simulink model "FUZZY_tsc_neurospora_model_leloup"  (R2015a)
settings: Solver=ode4  StartTime=0.0  StopTime=72  FixedStep=0.01  RelTol=1e-3
values from neighbouring files (symbols this model uses):
  daynight_on = 0    [ALL_neurospora_init.m]    (also in ALL_neurospora_sim_run.m; FUZZY_deg_neurospora_init.m; FUZZY_deg_neurospora_sim_run.m; FUZZY_tsc_neurospora_init.m)
  k_1 = 0.5    [ALL_neurospora_init.m]    (also in FUZZY_deg_neurospora_init.m; FUZZY_tsc_neurospora_init.m; FUZZY_tsc_tsl_neurospora_init.m; FUZZY_tsl_neurospora_init.m)
  k_2 = 0.6    [ALL_neurospora_init.m]    (also in FUZZY_deg_neurospora_init.m; FUZZY_tsc_neurospora_init.m; FUZZY_tsc_tsl_neurospora_init.m; FUZZY_tsl_neurospora_init.m)
  K_d = 0.13    [ALL_neurospora_init.m]    (also in FUZZY_deg_neurospora_init.m; FUZZY_tsc_neurospora_init.m; FUZZY_tsc_tsl_neurospora_init.m; FUZZY_tsl_neurospora_init.m)
  K_m = 0.5    [ALL_neurospora_init.m]    (also in FUZZY_deg_neurospora_init.m; FUZZY_tsc_neurospora_init.m; FUZZY_tsc_tsl_neurospora_init.m; FUZZY_tsl_neurospora_init.m)
  k_s = 0.5    [ALL_neurospora_init.m]    (also in FUZZY_deg_neurospora_init.m; FUZZY_tsc_neurospora_init.m; FUZZY_tsc_tsl_neurospora_init.m; FUZZY_tsl_neurospora_init.m)
  v_d = 1.4    [ALL_neurospora_init.m]    (also in FUZZY_deg_neurospora_init.m; FUZZY_tsc_neurospora_init.m; FUZZY_tsc_tsl_neurospora_init.m; FUZZY_tsl_neurospora_init.m)
  v_m = 0.505    [ALL_neurospora_init.m]    (also in FUZZY_deg_neurospora_init.m; FUZZY_tsc_neurospora_init.m; FUZZY_tsc_tsl_neurospora_init.m; FUZZY_tsl_neurospora_init.m)
libraries: fuzblock x1
settings Model: Creator=jureb  LastModifiedBy=jureb

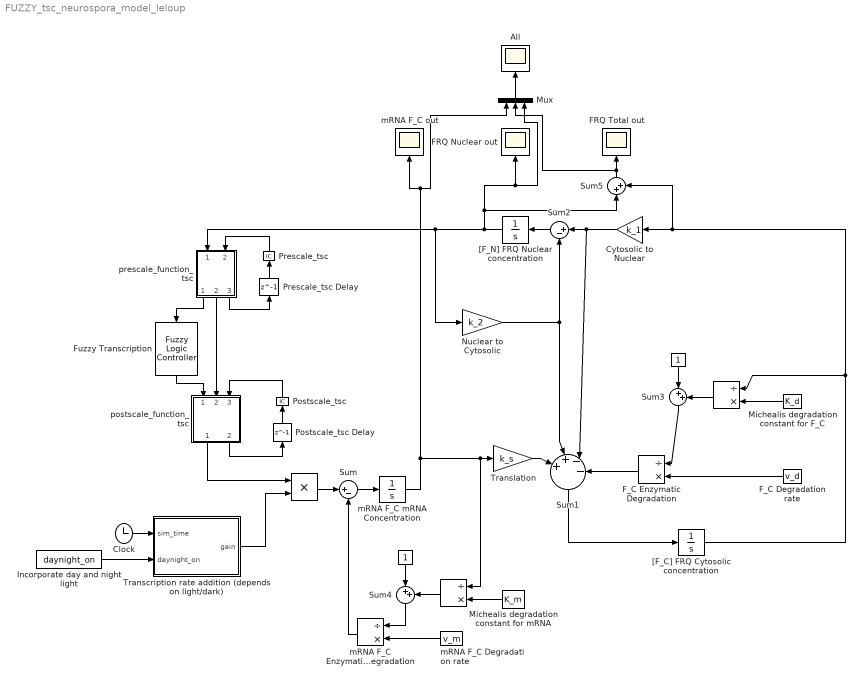
== system FUZZY_tsc_neurospora_model_leloup ==
  "    " : Product  Inputs=**
  " " : Product  Inputs=/*
  " " : Constant
  " " : Constant
  " " : Product  Inputs=/*
  All : Scope
      settings: TimeRange=71.999776  YMin=0  YMax=10  SaveName=All
  Clock : Clock
  Cytosolic to Nuclear : Gain  Gain=k_1
  FRQ Nuclear out : Scope
      settings: TimeRange=71.999776  YMin=0  YMax=4.5  SaveName=F_N
  FRQ Total out : Scope
      settings: TimeRange=71.999776  YMin=0.5  YMax=10  SaveName=F_FL_tsc
  F_C Degradation rate : Constant  Value=v_d
  F_C Enzymatic Degradation : Product  Inputs=/*
  Fuzzy Transcription : fuzblock/Fuzzy Logic  Controller  fis=tsc
  Incorporate day and night light : Constant  Value=daynight_on
  Michealis degradation constant for F_C : Constant  Value=K_d
  Michealis degradation constant for mRNA : Constant  Value=K_m
  Mux : Mux  Inputs=3
  Nuclear to Cytosolic : Gain  Gain=k_2
  Postscale_tsc : InitialCondition  Value=1.3
  Postscale_tsc Delay : Delay  DelayLength=1  InitialCondition=1
  Prescale_tsc : InitialCondition  Value=5
  Prescale_tsc Delay : Delay  DelayLength=1  InitialCondition=1  UseCircularBuffer=on
  Sum : Sum  Inputs=|+-
  Sum1 : Sum  Inputs=|+|+|-|-
  Sum2 : Sum  Inputs=|+-
  Sum3 : Sum  Inputs=|++
  Sum4 : Sum  Inputs=|++
  Sum5 : Sum  Inputs=|++
  Transcription rate addition (depends on light/dark) : MATLAB Function  TreatAsAtomicUnit=on
  Translation : Gain  Gain=k_s
  "[F_C] FRQ Cytosolic concentration " : Integrator  InitialCondition=1
  "[F_N] FRQ Nuclear concentration" : Integrator  InitialCondition=1
  mRNA F_C Degradation rate : Constant  Value=v_m
  mRNA F_C Enzymatic Degradation : Product  Inputs=/*
  mRNA F_C mRNA Concentration : Integrator  InitialCondition=1
  mRNA F_C out : Scope
      settings: TimeRange=71.999776  YMin=0  YMax=6  SaveName=mRNA
  postscale_function_tsc : MATLAB Function  TreatAsAtomicUnit=on
  prescale_function_tsc : MATLAB Function  TreatAsAtomicUnit=on
  wires:
  Sum/1 -> mRNA F_C mRNA Concentration/1
  mRNA F_C mRNA Concentration/1 -> " "/1, Translation/1, mRNA F_C out/1, Mux/1
  mRNA F_C Enzymatic Degradation/1 -> Sum/2
  "[F_N] FRQ Nuclear concentration"/1 -> prescale_function_tsc/1(input), Nuclear to Cytosolic/1, Mux/3, FRQ Nuclear out/1, Sum5/1
  Sum1/1 -> "[F_C] FRQ Cytosolic concentration "/1
  Cytosolic to Nuclear/1 -> Sum1/3, Sum2/1
  Sum2/1 -> "[F_N] FRQ Nuclear concentration"/1
  Nuclear to Cytosolic/1 -> Sum1/2, Sum2/2
  mRNA F_C Degradation rate/1 -> mRNA F_C Enzymatic Degradation/2
  " "/1 -> Sum4/1
  " "/1 -> Sum4/2
  Michealis degradation constant for mRNA/1 -> " "/2
  Sum4/1 -> mRNA F_C Enzymatic Degradation/1
  F_C Enzymatic Degradation/1 -> Sum1/4
  F_C Degradation rate/1 -> F_C Enzymatic Degradation/2
  " "/1 -> Sum3/1
  " "/1 -> Sum3/2
  Michealis degradation constant for F_C/1 -> " "/2
  Sum3/1 -> F_C Enzymatic Degradation/1
  Translation/1 -> Sum1/1
  Mux/1 -> All/1
  Sum5/1 -> Mux/2, FRQ Total out/1
  prescale_function_tsc/3(prescale_out) -> Prescale_tsc Delay/1
  Prescale_tsc/1 -> prescale_function_tsc/2(prescale_in)
  Postscale_tsc/1 -> postscale_function_tsc/3(postscale_in)
  postscale_function_tsc/2(postscale_out) -> Postscale_tsc Delay/1
  Prescale_tsc Delay/1 -> Prescale_tsc/1
  Postscale_tsc Delay/1 -> Postscale_tsc/1
  prescale_function_tsc/1(input_prescaled) -> Fuzzy Transcription/1
  postscale_function_tsc/1(output_postscaled) -> "    "/1
  Fuzzy Transcription/1 -> postscale_function_tsc/1(output)
  Incorporate day and night light/1 -> Transcription rate addition (depends on light/dark)/2(daynight_on)
  Clock/1 -> Transcription rate addition (depends on light/dark)/1(sim_time)
  Transcription rate addition (depends on light/dark)/1(gain) -> "    "/2
  prescale_function_tsc/2(prescale_changed) -> postscale_function_tsc/2(prescale_changed)
  "    "/1 -> Sum/1
  "[F_C] FRQ Cytosolic concentration "/1 -> Sum5/2, Cytosolic to Nuclear/1, " "/1

== matlab function FUZZY_tsc_neurospora_model_leloup/Transcription rate addition (depends on light//dark) ==
  data: sim_time input; gain output; daynight_on input
function gain = day_night(sim_time,daynight_on)

vs_day = 2;
vs_night = 1.6;

if daynight_on == 1
    if ((sim_time > 0 && sim_time < 12) || (sim_time > 24 && sim_time < 36) || (sim_time > 48 && sim_time < 60)) % DAY
        gain = vs_day/vs_night;
    else % NIGHT
        gain = 1;
    end
else % NO DIFFERENTIATION BETWEEN NIGHT AND DAY
    gain = 1;
end

== matlab function FUZZY_tsc_neurospora_model_leloup/prescale_function_tsc ==
  data: input input; input_prescaled output; prescale_changed output; prescale_in input; prescale_out output
function [input_prescaled, prescale_changed, prescale_out] = prescale(input, prescale_in)

prescale_out = prescale_in;
multiplier = 1.01;
prescale_changed = 0;

if (input >= 0.9*prescale_in)
    prescale_out = prescale_in*multiplier;
    prescale_changed = 1;
end

input_prescaled = input/prescale_out;

== matlab function FUZZY_tsc_neurospora_model_leloup/postscale_function_tsc ==
  data: output input; prescale_changed input; output_postscaled output; postscale_in input; postscale_out output
function [output_postscaled, postscale_out] = postscale(output, prescale_changed, postscale_in)

postscale_out = postscale_in;
multiplier = 1.01;

if (prescale_changed == 1)
    postscale_out = postscale_out*multiplier;
end

output_postscaled = output*postscale_out;
